simulink model "assignment_b4_simulink"  (Simulink 8.1)
settings: Solver=ode45  StartTime=0.0  StopTime=10.0  RelTol=1e-3
settings Model: Creator=USER  LastModifiedBy=USER
settings DataIOCC: SignalLoggingSaveFormat=Dataset
settings OptimizationCC: ExpressionDepthLimit=128
settings DebuggingCC: FcnCallInpInsideContextMsg=EnableAllAsError
settings GRTTargetCC: CombineOutputUpdateFcns=on  GRTInterface=off

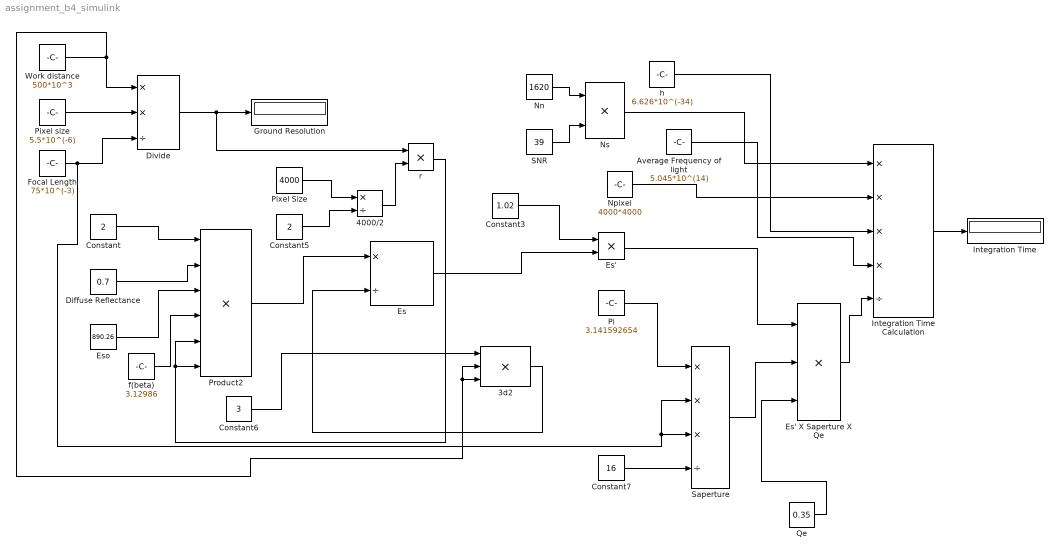
== system assignment_b4_simulink ==
  3d2 : Product  Inputs=3
  4000/2 : Product  Inputs=*/
  Average Frequency of light : Constant  Value=5.045*10^(14)
  Constant : Constant  Value=2
  Constant3 : Constant  Value=1.02
  Constant5 : Constant  Value=2
  Constant6 : Constant  Value=3
  Constant7 : Constant  Value=16
  Diffuse Reflectance : Constant  Value=0.7
  Divide : Product  Inputs=**/
  Es : Product  Inputs=*/
  Es' : Product
  Es' X Saperture X Qe : Product  Inputs=3
  Eso : Constant  Value=890.26
  Focal Length : Constant  Value=75*10^(-3)
  Ground Resolution : Display
  Integration Time : Display
  Integration Time Calculation : Product  Inputs=****/
  Nn : Constant  Value=1620
  Npixel : Constant  Value=4000*4000
  Ns : Product
  Pi : Constant  Value=3.141592654
  Pixel Size : Constant  Value=4000
  Pixel size : Constant  Value=5.5*10^(-6)
  Product2 : Product  Inputs=6
  Qe : Constant  Value=0.35
  SNR : Constant  Value=39
  Saperture : Product  Inputs=***/
  "Work distance " : Constant  Value=500*10^3
  f(beta) : Constant  Value=3.12986
  h : Constant  Value=6.626*10^(-34)
  r : Product
  wires:
  "Work distance "/1 -> Divide/1, 3d2/3, 3d2/2
  Pixel size/1 -> Divide/2
  Focal Length/1 -> Saperture/2, Saperture/3, Divide/3
  Divide/1 -> r/1, Ground Resolution/1
  Pixel Size/1 -> 4000/2/1
  Constant5/1 -> 4000/2/2
  4000/2/1 -> r/2
  Constant3/1 -> Es'/1
  Pi/1 -> Saperture/1
  Constant7/1 -> Saperture/4
  Constant/1 -> Product2/1
  Diffuse Reflectance/1 -> Product2/2
  Eso/1 -> Product2/3
  Nn/1 -> Ns/1
  SNR/1 -> Ns/2
  Es'/1 -> Es' X Saperture X Qe/1
  Saperture/1 -> Es' X Saperture X Qe/2
  Qe/1 -> Es' X Saperture X Qe/3
  Ns/1 -> Integration Time Calculation/1
  Npixel/1 -> Integration Time Calculation/2
  h/1 -> Integration Time Calculation/3
  Average Frequency of light/1 -> Integration Time Calculation/4
  Es' X Saperture X Qe/1 -> Integration Time Calculation/5
  Integration Time Calculation/1 -> Integration Time/1
  f(beta)/1 -> Product2/4
  r/1 -> Product2/6, Product2/5
  Product2/1 -> Es/1
  3d2/1 -> Es/2
  Es/1 -> Es'/2
  Constant6/1 -> 3d2/1
